simulink model "ImuCalibrator"  (R2018a)
settings: Solver=FixedStepDiscrete  StartTime=0.0  StopTime=inf  FixedStep=1/Fss  RelTol=1e-3
PreLoadFcn:
  | modelDef = getModelDef();
  | Fss = 1;  % nominal IMU sampling rate
  | 
  | gyroCalBiases = [0;0;0];
  | gyroCalMatrix = eye(3);
  | gyroGsensMatrix = zeros(3,3);
  | 
  | accelCalBiases = [0;0;0];
  | accelCalMatrix = eye(3);
  | 
  | imuPar = getImuPar('lmvpUncalibrated');
  | 
  | lastUsedMgyr = zeros(3,3);
undefined symbols (not defined in the file or in its folder): numStates
libraries: simulink x5, vrlib x5, dspinverses x4, dspsigops x2, dspindex x2, dspstat3 x1, simulink_extras x1, dspmtrx3 x1, dspsnks4 x1, dspsrcs4 x1, dspswit3 x1
(part 1 of 2)
settings Model: Creator=Eric  LastModifiedBy=efoxlin
settings OptimizationCC: DefaultParameterBehavior=Inlined  InlineInvariantSignals=on
settings DebuggingCC: UnconnectedOutputMsg=none
settings RTWCC: Toolchain=Microsoft Visual C++ 2017 v15.0 | nmake (64-bit Windows)  BuildConfiguration=Faster Runs
settings GRTTargetCC: MatFileLogging=off  SupportNonFinite=off

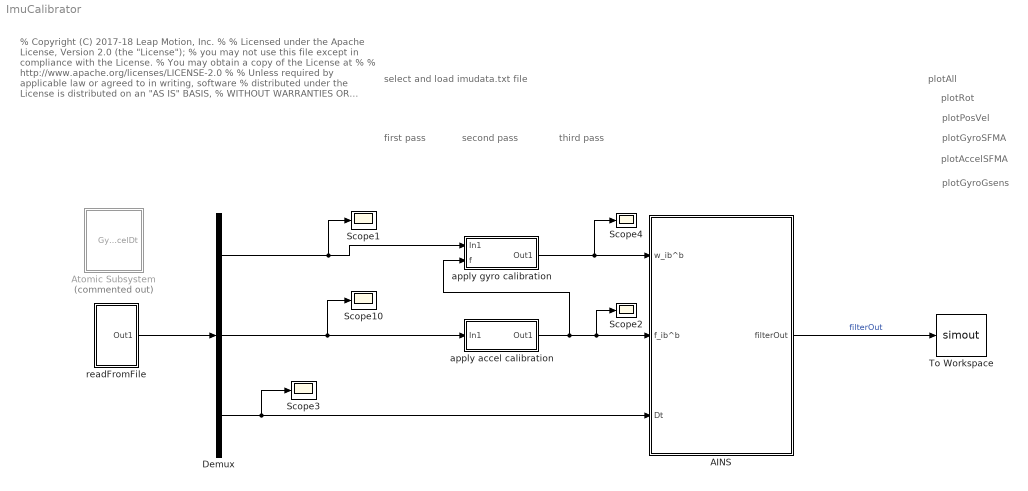
== system ImuCalibrator ==
  note: % Copyright (C) 2017-18 Leap Motion, Inc.
      | %
      | %    Licensed under the Apache License, Version 2.0 (the "License");
      | %    you may not use this file except in compliance with the License.
      | %    You may obtain a copy of the License at
      | %
      | %        http://www.apache.org/licenses/LICENSE-2.0
      | %
      | %    Unless required by applicable law or agreed to in writing, software
      | %    distributed under the License is distributed on an "AS IS" BASIS,
      | %    WITHOUT WARRANTIES OR CONDITIONS OF ANY KIND, either express or implied.
      | %    See the License for the specific language governing permissions and
      | %    limitations under the License.
      | % Author: Eric Foxlin
  note: select and load imudata.txt file
  note: second pass
  note: first pass
  note: plotAccelSFMA
  note: plotGyroSFMA
  note: plotAll
  note: plotPosVel
  note: plotRot
  note: plotGyroGsens
  note: third pass
  AINS : Subsystem  TreatAsAtomicUnit=on
  Atomic Subsystem : Subsystem  Commented=on  TreatAsAtomicUnit=on
  Demux : Demux  Outputs=[3 3 1]
  Scope{1..4,10} (5 alike) : Scope
  To Workspace : ToWorkspace  VariableName=simout  SaveFormat=Timeseries  SampleTime=-1
      settings: Save2DSignal=2-D array (concatenate along first dimension)
  apply accel calibration : Subsystem  TreatAsAtomicUnit=on
  apply gyro calibration : Subsystem  TreatAsAtomicUnit=on
  readFromFile : Subsystem
  wires:
  Demux/3 -> Scope3/1, AINS/3(Dt)
  Demux/2 -> Scope10/1, apply accel calibration/1(In1)
  apply gyro calibration/1(Out1) -> AINS/1(w_ib^b), Scope4/1
  apply accel calibration/1(Out1) -> AINS/2(f_ib^b), Scope2/1, apply gyro calibration/2(f)
  Demux/1 -> apply gyro calibration/1(In1), Scope1/1
  readFromFile/1(Out1) -> Demux/1
  AINS/1(filterOut) -> To Workspace/1  "filterOut"

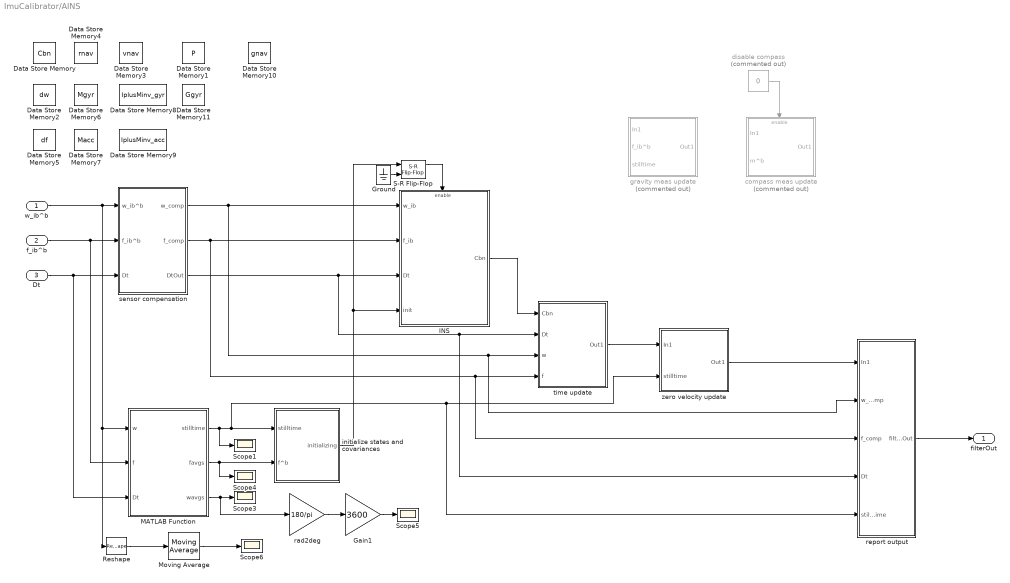
== system ImuCalibrator/AINS ==
  w_ib^b : Inport  Unit=rad/s
  f_ib^b : Inport  Port=2  Unit=m/s^2  PortDimensions=3
  Dt : Inport  Port=3  Unit=rad/s
  Data Store Memory : DataStoreMemory  DataStoreName=Cbn  ReadBeforeWriteMsg=warning  WriteAfterWriteMsg=warning  WriteAfterReadMsg=warning  InitialValue=eye(3)  VectorParams1D=off  ShowAdditionalParam=off
  Data Store Memory1 : DataStoreMemory  DataStoreName=P  ReadBeforeWriteMsg=warning  WriteAfterWriteMsg=warning  WriteAfterReadMsg=warning  InitialValue=eye(modelDef.numStates)*1e-12  ShowAdditionalParam=off
  Data Store Memory10 : DataStoreMemory  DataStoreName=gnav  ReadBeforeWriteMsg=warning  WriteAfterWriteMsg=warning  WriteAfterReadMsg=warning  InitialValue=[0;0; 9.8065]  VectorParams1D=off  ShowAdditionalParam=off
  Data Store Memory11 : DataStoreMemory  DataStoreName=Ggyr  ReadBeforeWriteMsg=warning  WriteAfterWriteMsg=warning  WriteAfterReadMsg=warning  InitialValue=zeros(3,3)  VectorParams1D=off  ShowAdditionalParam=off
  Data Store Memory2 : DataStoreMemory  DataStoreName=dw  ReadBeforeWriteMsg=warning  WriteAfterWriteMsg=warning  WriteAfterReadMsg=warning  InitialValue=[0;0;0]  VectorParams1D=off  ShowAdditionalParam=off
  Data Store Memory3 : DataStoreMemory  DataStoreName=vnav  ReadBeforeWriteMsg=warning  WriteAfterWriteMsg=warning  WriteAfterReadMsg=warning  InitialValue=[0;0;0]  VectorParams1D=off  ShowAdditionalParam=off
  Data Store Memory4 : DataStoreMemory  DataStoreName=rnav  ReadBeforeWriteMsg=warning  WriteAfterWriteMsg=warning  WriteAfterReadMsg=warning  InitialValue=[0;0;0]  VectorParams1D=off  ShowAdditionalParam=off
  Data Store Memory5 : DataStoreMemory  DataStoreName=df  ReadBeforeWriteMsg=warning  WriteAfterWriteMsg=warning  WriteAfterReadMsg=warning  InitialValue=[0;0;0]  VectorParams1D=off  ShowAdditionalParam=off
  Data Store Memory6 : DataStoreMemory  DataStoreName=Mgyr  ReadBeforeWriteMsg=warning  WriteAfterWriteMsg=warning  WriteAfterReadMsg=warning  InitialValue=zeros(3,3)  VectorParams1D=off  ShowAdditionalParam=off
  Data Store Memory7 : DataStoreMemory  DataStoreName=Macc  ReadBeforeWriteMsg=warning  WriteAfterWriteMsg=warning  WriteAfterReadMsg=warning  InitialValue=zeros(3,3)  VectorParams1D=off  ShowAdditionalParam=off
  Data Store Memory8 : DataStoreMemory  DataStoreName=IplusMinv_gyr  ReadBeforeWriteMsg=warning  WriteAfterWriteMsg=warning  WriteAfterReadMsg=warning  InitialValue=eye(3)  VectorParams1D=off  ShowAdditionalParam=off
  Data Store Memory9 : DataStoreMemory  DataStoreName=IplusMinv_acc  ReadBeforeWriteMsg=warning  WriteAfterWriteMsg=warning  WriteAfterReadMsg=warning  InitialValue=eye(3)  VectorParams1D=off  ShowAdditionalParam=off
  Gain1 : Gain  Gain=3600
  Ground : Ground
  INS : Subsystem  Priority=2
  MATLAB Function : MATLAB Function  TreatAsAtomicUnit=on
  Moving Average : dspstat3/Moving Average  Method=Sliding window  ForgettingFactorPort=off  SpecifyWindowLength=on  WindowLength=1000  ForgettingFactor=0.9  SimulateUsing=Code generation
  Reshape : Reshape  OutputDimensionality=Row vector (2-D)
  S-R Flip-Flop : simulink_extras/Flip Flops/S-R Flip-Flop  initial_condition=0
  Scope{1,3..6} (5 alike) : Scope
  compass meas update : Subsystem  Commented=on  TreatAsAtomicUnit=on
  disable compass : Constant  Commented=on  Value=0
  gravity meas update : Subsystem  Commented=on  TreatAsAtomicUnit=on
  initialize states and covariances : Subsystem  Priority=1  TreatAsAtomicUnit=on
  rad2deg : Gain  Gain=180/pi
  report output : Subsystem  Priority=10  TreatAsAtomicUnit=on
  sensor compensation : Subsystem
  time update : Subsystem  Priority=3  TreatAsAtomicUnit=on
  zero velocity update : Subsystem  Priority=4  TreatAsAtomicUnit=on
  filterOut : Outport
  wires:
  time update/1(Out1) -> zero velocity update/1(In1)
  disable compass/1 -> compass meas update/Enable
  MATLAB Function/1(stilltime) -> Scope1/1, report output/5(stilltime), zero velocity update/2(stilltime), initialize states and covariances/1(stilltime)
  MATLAB Function/2(favgs) -> Scope4/1, initialize states and covariances/2(f^b)
  zero velocity update/1(Out1) -> report output/1(In1)
  sensor compensation/1(w_comp) -> report output/2(w_comp), time update/3(w), INS/1(w_ib)
  INS/1(Cbn) -> time update/1(Cbn)
  sensor compensation/3(DtOut) -> report output/4(Dt), time update/2(Dt), INS/3(Dt)
  sensor compensation/2(f_comp) -> INS/2(f_ib), report output/3(f_comp), time update/4(f)
  f_ib^b/1 -> MATLAB Function/2(f), sensor compensation/2(f_ib^b)
  w_ib^b/1 -> MATLAB Function/1(w), Reshape/1, sensor compensation/1(w_ib^b)
  Dt/1 -> MATLAB Function/3(Dt), sensor compensation/3(Dt)
  initialize states and covariances/1(initializing) -> INS/4(init), S-R Flip-Flop/1
  MATLAB Function/3(wavgs) -> rad2deg/1, Scope3/1
  rad2deg/1 -> Gain1/1
  Gain1/1 -> Scope5/1
  Moving Average/1 -> Scope6/1
  Reshape/1 -> Moving Average/1
  S-R Flip-Flop/1 -> INS/Enable
  report output/1(filterOut) -> filterOut/1
  Ground/1 -> S-R Flip-Flop/2

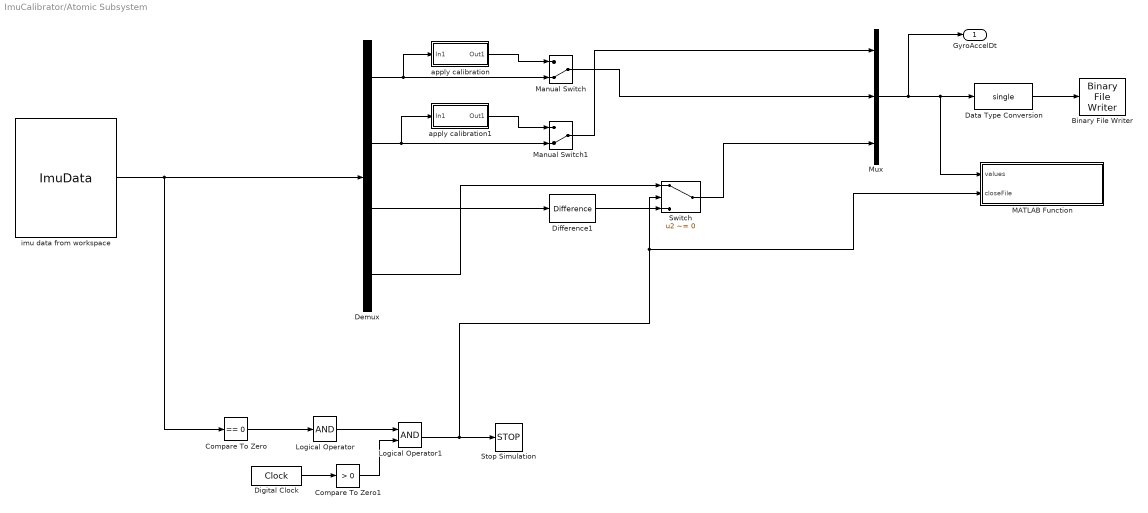
== system ImuCalibrator/Atomic Subsystem ==
  Binary File Writer : dspsnks4/Binary File Writer  Filename=GyroAccelDtFloat32.bin  HeaderStructure=struct([])  SimulateUsing=Code generation
      settings: SourceProductName=DSP System Toolbox  SourceProductBaseCode=DS
  Compare To Zero : simulink/Logic and Bit Operations/Compare To Zero  relop===  OutDataTypeStr=boolean
  Compare To Zero1 : simulink/Logic and Bit Operations/Compare To Zero  relop=>  OutDataTypeStr=boolean
  Data Type Conversion : DataTypeConversion  OutDataTypeStr=single
  Demux : Demux  Outputs=[ 3 3 1 1]
  Difference1 : simulink/Discrete/Difference  ICPrevInput=0.0  OutMin=[]  OutMax=[]  OutDataType=fixdt(1, 16)  OutScaling=2^-10  DoSatur=off
  Digital Clock : DigitalClock  SampleTime=1/Fss
  Logical Operator : Logic  Inputs=1  AllPortsSameDT=off  OutDataTypeStr=boolean
  Logical Operator1 : Logic  AllPortsSameDT=off  OutDataTypeStr=boolean
  MATLAB Function : MATLAB Function  TreatAsAtomicUnit=on
  Manual Switch : ManualSwitch  CurrentSetting=0
  Manual Switch1 : ManualSwitch  CurrentSetting=0
  Mux : Mux  Inputs=[3 3 1]
  Stop Simulation : Stop
  Switch : Switch  Criteria=u2 ~= 0  Threshold=0.5
  apply calibration : Subsystem  TreatAsAtomicUnit=on
  apply calibration1 : Subsystem  TreatAsAtomicUnit=on
  imu data from workspace : FromWorkspace  VariableName=ImuData  SampleTime=1/Fss  Interpolate=off  OutputAfterFinalValue=Setting to zero
  GyroAccelDt : Outport
  wires:
  imu data from workspace/1 -> Compare To Zero/1, Demux/1
  Demux/1 -> Manual Switch/2, apply calibration/1(In1)
  Demux/2 -> Manual Switch1/2, apply calibration1/1(In1)
  Compare To Zero/1 -> Logical Operator/1
  Logical Operator/1 -> Logical Operator1/1
  Manual Switch/1 -> Mux/2
  apply calibration/1(Out1) -> Manual Switch/1
  apply calibration1/1(Out1) -> Manual Switch1/1
  Manual Switch1/1 -> Mux/1
  Logical Operator1/1 -> MATLAB Function/2(closeFile), Switch/2, Stop Simulation/1
  Digital Clock/1 -> Compare To Zero1/1
  Compare To Zero1/1 -> Logical Operator1/2
  Demux/3 -> Difference1/1
  Difference1/1 -> Switch/3
  Switch/1 -> Mux/3
  Demux/4 -> Switch/1
  Mux/1 -> GyroAccelDt/1, MATLAB Function/1(values), Data Type Conversion/1
  Data Type Conversion/1 -> Binary File Writer/1

== system ImuCalibrator/apply accel calibration ==
  In1 : Inport
  Accel SFMA matrix    ameas = M*atrue : Constant  Value=accelCalMatrix  VectorParams1D=off
  "Accel SFMA matrix, column-major1" : Constant  Value="[0.9973\t0.0126\t0.0025\t0.0004\t1.0177\t0.003\t0.0064\t0.0308\t1.0224]"  VectorParams1D=off
  Matrix Multiply : Product  Multiplication=Matrix(*)
  Sum : Sum  Inputs=|+-
  "bias, mg" : Constant  Value=accelCalBiases  VectorParams1D=off
  Out1 : Outport
  wires:
  In1/1 -> Sum/1
  Matrix Multiply/1 -> Out1/1
  Sum/1 -> Matrix Multiply/2
  "bias, mg"/1 -> Sum/2
  Accel SFMA matrix    ameas = M*atrue/1 -> Matrix Multiply/1

== system ImuCalibrator/apply gyro calibration ==
  In1 : Inport
  f : Inport  Port=2
  Accel SFMA matrix    ameas = M*atrue : Constant  Value=gyroCalMatrix  VectorParams1D=off
  Accel SFMA matrix    ameas = M*atrue1 : Constant  Value=gyroGsensMatrix  VectorParams1D=off
  "Accel SFMA matrix, column-major1" : Constant  Value="[0.9973\t0.0126\t0.0025\t0.0004\t1.0177\t0.003\t0.0064\t0.0308\t1.0224]"  VectorParams1D=off
  Matrix Multiply : Product  Multiplication=Matrix(*)
  Matrix Multiply1 : Product  Multiplication=Matrix(*)
  Sum : Sum  Inputs=|+-
  Sum1 : Sum  Inputs=|+-
  "bias, mg" : Constant  Value=gyroCalBiases  VectorParams1D=off
  Out1 : Outport
  wires:
  Accel SFMA matrix    ameas = M*atrue/1 -> Matrix Multiply/1
  "bias, mg"/1 -> Sum/2
  Sum/1 -> Matrix Multiply/2
  Matrix Multiply/1 -> Out1/1
  In1/1 -> Sum1/1
  Sum1/1 -> Sum/1
  Matrix Multiply1/1 -> Sum1/2
  f/1 -> Matrix Multiply1/2
  Accel SFMA matrix    ameas = M*atrue1/1 -> Matrix Multiply1/1

== system ImuCalibrator/readFromFile ==
  Binary File Reader : dspsrcs4/Binary File Reader  Commented=on  Filename=GyroAccelDtFloat32.bin  HeaderStructure=struct([])  DataType=single  SamplesPerFrame=1  IsDataComplex=off  NumChannels=7  OutputEOF=on  SampleTime=1/Fss  SimulateUsing=Code generation
      settings: SourceProductName=DSP System Toolbox  SourceProductBaseCode=DS
  Counter : dspswit3/Counter  Direction=Up  CountEvent=Free running  CounterSize=User defined  MaxCount=4095  InitialCount=0  Output=Hit  HitValue=32  ResetInput=off  SamplesPerFrame=1  Ts=1/Fss  CntDtype=double  HitDtype=Logical
  Data Type Conversion : DataTypeConversion  OutDataTypeStr=double
  MATLAB Function1 : MATLAB Function  Commented=on  TreatAsAtomicUnit=on
  Reshape : Reshape  OutputDimensionality=Column vector (2-D)
  Stop Simulation : Stop
  printTime : Subsystem
  readImuData : Subsystem
  Out1 : Outport
  wires:
  Reshape/1 -> Data Type Conversion/1
  readImuData/1(GyrosAccelsDt) -> Reshape/1
  readImuData/2(EOF) -> Stop Simulation/1
  Data Type Conversion/1 -> Out1/1
  Counter/1 -> printTime/Enable

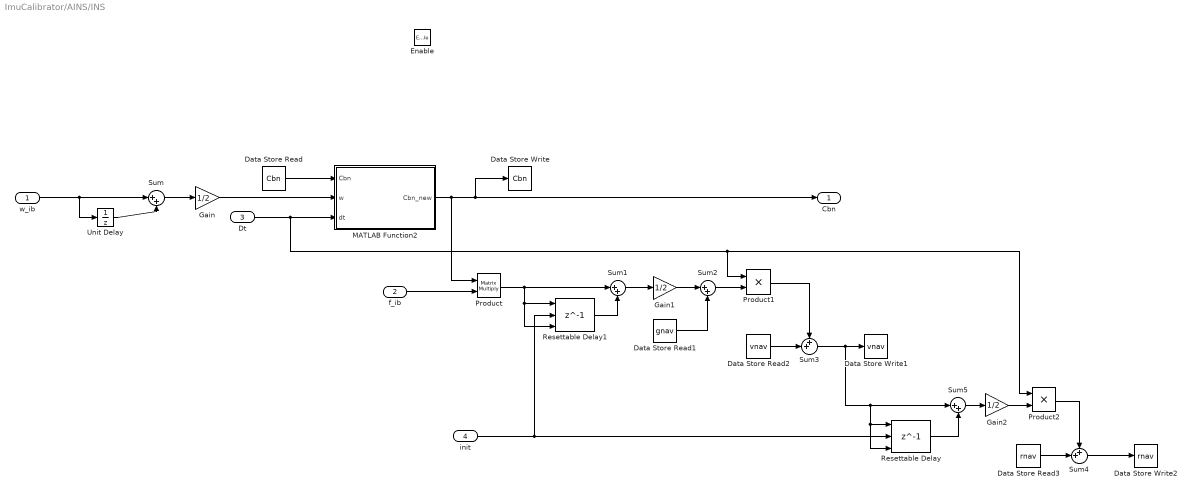
== system ImuCalibrator/AINS/INS ==
  w_ib : Inport
  f_ib : Inport  Port=2
  Dt : Inport  Port=3
  init : Inport  Port=4
  Enable : EnablePort
  Data Store Read : DataStoreRead  DataStoreName=Cbn
  Data Store Read1 : DataStoreRead  DataStoreName=gnav
  Data Store Read2 : DataStoreRead  DataStoreName=vnav
  Data Store Read3 : DataStoreRead  DataStoreName=rnav
  Data Store Write : DataStoreWrite  DataStoreName=Cbn
  Data Store Write1 : DataStoreWrite  DataStoreName=vnav
  Data Store Write2 : DataStoreWrite  DataStoreName=rnav
  Gain : Gain  Gain=1/2
  Gain1 : Gain  Gain=1/2
  Gain2 : Gain  Gain=1/2
  MATLAB Function2 : MATLAB Function  TreatAsAtomicUnit=on
  Product : Product  Multiplication=Matrix(*)
  Product1 : Product
  Product2 : Product
  Resettable Delay : Delay  DelayLength=1  InitialConditionSource=Input port  ExternalReset=Level
      settings: InputPortMap=u0,r5,p4
  Resettable Delay1 : Delay  DelayLength=1  InitialConditionSource=Input port  ExternalReset=Level
      settings: InputPortMap=u0,r5,p4
  Sum{,1..2,5} (4 alike) : Sum  Inputs=|++
  Sum3 : Sum  Inputs=++|
  Sum4 : Sum  Inputs=++|
  Unit Delay : UnitDelay  SampleTime=-1
  Cbn : Outport
  wires:
  Dt/1 -> Product2/1, Product1/1, MATLAB Function2/3(dt)
  Data Store Read/1 -> MATLAB Function2/1(Cbn)
  w_ib/1 -> Unit Delay/1, Sum/1
  MATLAB Function2/1(Cbn_new) -> Product/1, Cbn/1, Data Store Write/1
  Unit Delay/1 -> Sum/2
  Sum/1 -> Gain/1
  Gain/1 -> MATLAB Function2/2(w)
  f_ib/1 -> Product/2
  Data Store Read1/1 -> Sum2/2
  Sum2/1 -> Product1/2
  Product/1 -> Resettable Delay1/3, Resettable Delay1/1, Sum1/1
  Sum1/1 -> Gain1/1
  Gain1/1 -> Sum2/1
  Data Store Read2/1 -> Sum3/2
  Product1/1 -> Sum3/1
  Data Store Read3/1 -> Sum4/2
  Sum4/1 -> Data Store Write2/1
  Sum5/1 -> Gain2/1
  Sum3/1 -> Resettable Delay/3, Resettable Delay/1, Sum5/1, Data Store Write1/1
  Gain2/1 -> Product2/2
  Resettable Delay/1 -> Sum5/2
  init/1 -> Resettable Delay1/2, Resettable Delay/2
  Resettable Delay1/1 -> Sum1/2
  Product2/1 -> Sum4/1

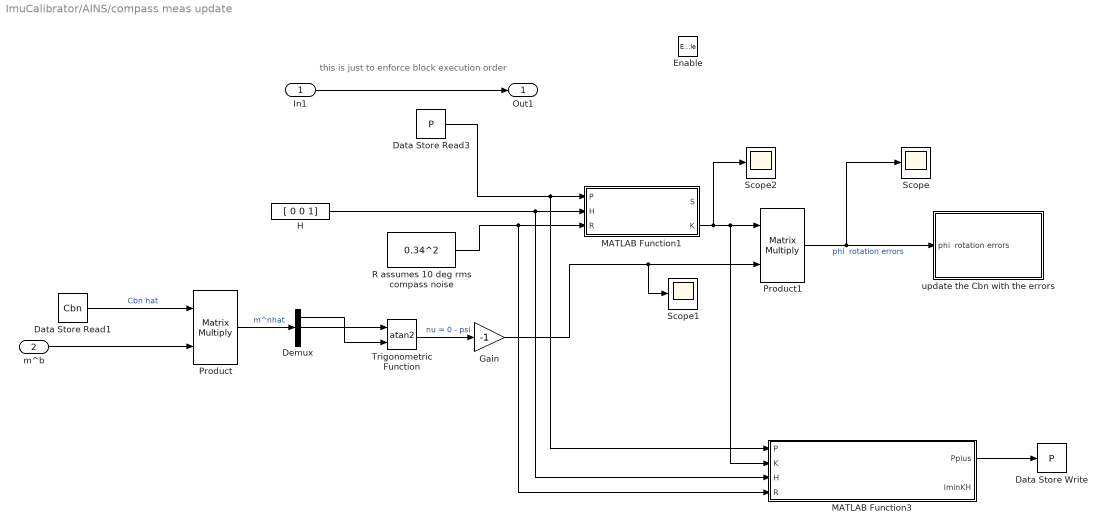
== system ImuCalibrator/AINS/compass meas update ==
  note: this is just to enforce block execution order
  In1 : Inport
  m^b : Inport  Port=2
  Enable : EnablePort
  Data Store Read1 : DataStoreRead  DataStoreName=Cbn
  Data Store Read3 : DataStoreRead  DataStoreName=P
  Data Store Write : DataStoreWrite  DataStoreName=P
  Demux : Demux  Outputs=3
  Gain : Gain  Gain=-1
  H : Constant  Value=[ 0 0 1]  VectorParams1D=off
  MATLAB Function1 : MATLAB Function  TreatAsAtomicUnit=on
  MATLAB Function3 : MATLAB Function  TreatAsAtomicUnit=on
  Product : Product  Multiplication=Matrix(*)
  Product1 : Product  Multiplication=Matrix(*)
  R assumes 10 deg rms compass noise : Constant  Value=0.34^2
  Scope : Scope
  Scope1 : Scope
  Scope2 : Scope
  Trigonometric Function : Trigonometry  Operator=atan2
  update the Cbn with the errors : Subsystem
  Out1 : Outport
  wires:
  Product1/1 -> update the Cbn with the errors/1(phi  rotation errors), Scope/1  "phi  rotation errors"
  R assumes 10 deg rms compass noise/1 -> MATLAB Function1/3(R), MATLAB Function3/4(R)
  Data Store Read3/1 -> MATLAB Function1/1(P), MATLAB Function3/1(P)
  m^b/1 -> Product/2
  MATLAB Function3/1(Pplus) -> Data Store Write/1
  MATLAB Function1/2(K) -> Product1/1, MATLAB Function3/2(K), Scope2/1
  Trigonometric Function/1 -> Gain/1  "nu = 0 - psi"
  Product/1 -> Demux/1  "m^nhat"
  Data Store Read1/1 -> Product/1  "Cbn hat"
  In1/1 -> Out1/1
  Demux/2 -> Trigonometric Function/1
  Demux/1 -> Trigonometric Function/2
  H/1 -> MATLAB Function1/2(H), MATLAB Function3/3(H)
  Gain/1 -> Product1/2, Scope1/1

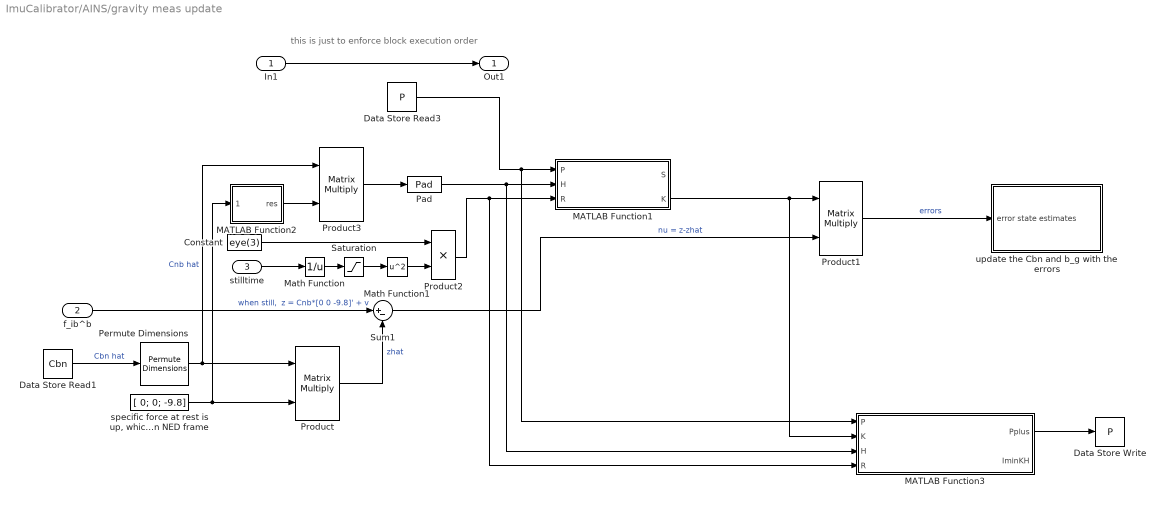
== system ImuCalibrator/AINS/gravity meas update ==
  note: this is just to enforce block execution order
  In1 : Inport
  f_ib^b : Inport  Port=2
  stilltime : Inport  Port=3
  Constant : Constant  Value=eye(3)
  Data Store Read1 : DataStoreRead  DataStoreName=Cbn
  Data Store Read3 : DataStoreRead  DataStoreName=P
  Data Store Write : DataStoreWrite  DataStoreName=P
  MATLAB Function1 : MATLAB Function  TreatAsAtomicUnit=on
  MATLAB Function2 : MATLAB Function  TreatAsAtomicUnit=on
  MATLAB Function3 : MATLAB Function  TreatAsAtomicUnit=on
  Math Function : Math  Operator=reciprocal  SaturateOnIntegerOverflow=on
  Math Function1 : Math  Operator=square  SaturateOnIntegerOverflow=on
  Pad : dspsigops/Pad  padAlong=Rows  dimsToPad=1  valSrc=Specify via dialog  padVal=0  spec=Output size  padNumOutRowsSpecMethod=User-specified  numOutRows=1  padNumOutColsSpecMethod=User-specified  numOutCols=numStates  isVarDimsMode=off  padBeginning=0  padEnd=0  outSizeMode=User-specified  outSize=1  padSigAt=End  trunc_flag=None  roundingMode=Floor  overflowMode=off  truncOrWrapMode=Truncate  wrap_flag=None
      settings: SourceProductName=DSP System Toolbox  SourceProductBaseCode=DS
  Permute Dimensions : PermuteDimensions
  Product : Product  Multiplication=Matrix(*)
  Product1 : Product  Multiplication=Matrix(*)
  Product2 : Product
  Product3 : Product  Multiplication=Matrix(*)
  Saturation : Saturate  UpperLimit=9.8*4  LowerLimit=1
  Sum1 : Sum  Inputs=|+-
  "specific force at rest is up, which is -z in NED frame" : Constant  Value=[ 0; 0; -9.8]
  update the Cbn and b_g with the errors : Subsystem
  Out1 : Outport
  wires:
  In1/1 -> Out1/1
  f_ib^b/1 -> Sum1/1  "when still,  z = Cnb*[0 0 -9.8]' + v"
  Data Store Read1/1 -> Permute Dimensions/1  "Cbn hat"
  Permute Dimensions/1 -> Product3/1, Product/1  "Cnb hat"
  Product/1 -> Sum1/2  "zhat"
  Sum1/1 -> Product1/2  "nu = z-zhat"
  MATLAB Function3/1(Pplus) -> Data Store Write/1
  Product3/1 -> Pad/1
  "specific force at rest is up, which is -z in NED frame"/1 -> MATLAB Function2/1(inp_vr), Product/2
  MATLAB Function2/1(res) -> Product3/2
  Data Store Read3/1 -> MATLAB Function3/1(P), MATLAB Function1/1(P)
  Product2/1 -> MATLAB Function3/4(R), MATLAB Function1/3(R)
  Product1/1 -> update the Cbn and b_g with the errors/1(" error state estimates")  "errors"
  Constant/1 -> Product2/1
  Math Function/1 -> Saturation/1
  Saturation/1 -> Math Function1/1
  stilltime/1 -> Math Function/1
  Math Function1/1 -> Product2/2
  Pad/1 -> MATLAB Function3/3(H), MATLAB Function1/2(H)
  MATLAB Function1/2(K) -> Product1/1, MATLAB Function3/2(K)

== system ImuCalibrator/AINS/initialize states and covariances ==
  stilltime : Inport
  f^b : Inport  Port=2
  Compare To Constant : simulink/Logic and Bit Operations/Compare To Constant  relop=>  const=1.0  OutDataTypeStr=boolean
  Data Store Memory : DataStoreMemory  DataStoreName=INITIALIZED  ReadBeforeWriteMsg=warning  WriteAfterWriteMsg=warning  WriteAfterReadMsg=warning  ShowAdditionalParam=off
  Data Store Read : DataStoreRead  DataStoreName=INITIALIZED
  INITIALIZED = 1 : Subsystem
  Logical Operator : Logic  AllPortsSameDT=off  OutDataTypeStr=boolean
  Logical Operator1 : Logic  Operator=NOT  Inputs=1  IconShape=distinctive  AllPortsSameDT=off  OutDataTypeStr=boolean
  calc Cbn : Subsystem  TreatAsAtomicUnit=on
  set P : Subsystem
  set states : Subsystem  TreatAsAtomicUnit=on
  initializing : Outport
  wires:
  Compare To Constant/1 -> Logical Operator/2
  stilltime/1 -> Compare To Constant/1
  Data Store Read/1 -> Logical Operator1/1
  Logical Operator1/1 -> Logical Operator/1
  f^b/1 -> calc Cbn/1(f^b)
  calc Cbn/2(Cbn) -> set states/1(Cbn)
  INITIALIZED = 1/1(Out1) -> initializing/1
  Logical Operator/1 -> calc Cbn/Enable
  calc Cbn/1(Out1) -> set states/Enable
  set states/1(Out1) -> set P/Enable
  set P/1(Out1) -> INITIALIZED = 1/Enable

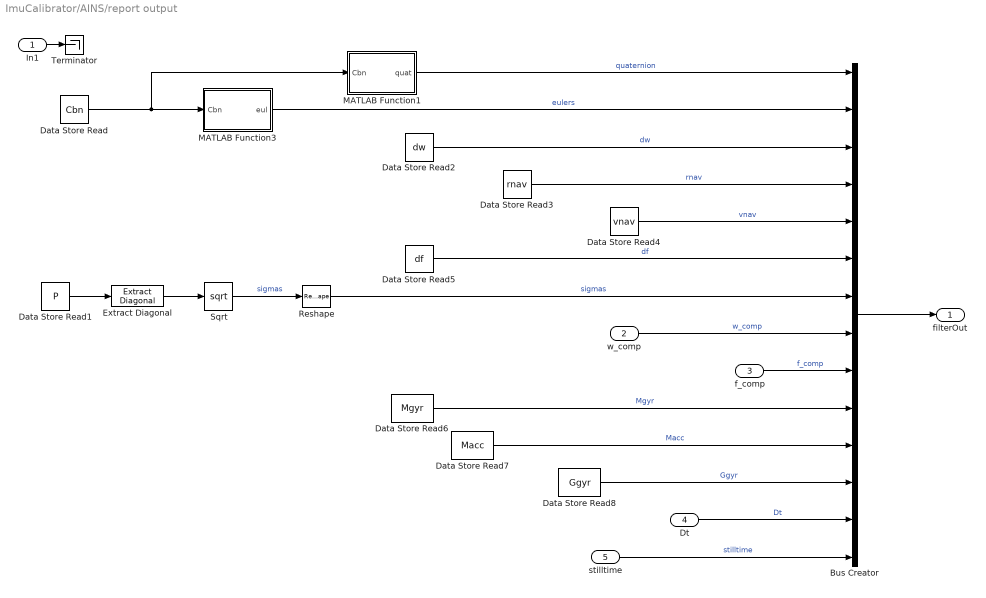
== system ImuCalibrator/AINS/report output ==
  In1 : Inport
  w_comp : Inport  Port=2
  f_comp : Inport  Port=3
  Dt : Inport  Port=4
  stilltime : Inport  Port=5
  Bus Creator : BusCreator  Inputs=14
  Data Store Read : DataStoreRead  DataStoreName=Cbn
  Data Store Read1 : DataStoreRead  DataStoreName=P
  Data Store Read2 : DataStoreRead  DataStoreName=dw
  Data Store Read3 : DataStoreRead  DataStoreName=rnav
  Data Store Read4 : DataStoreRead  DataStoreName=vnav
  Data Store Read5 : DataStoreRead  DataStoreName=df
  Data Store Read6 : DataStoreRead  DataStoreName=Mgyr
  Data Store Read7 : DataStoreRead  DataStoreName=Macc
  Data Store Read8 : DataStoreRead  DataStoreName=Ggyr
  Extract Diagonal : dspmtrx3/Extract Diagonal
      settings: SourceProductName=DSP System Toolbox  SourceProductBaseCode=DS
  MATLAB Function1 : MATLAB Function  TreatAsAtomicUnit=on
  MATLAB Function3 : MATLAB Function  TreatAsAtomicUnit=on
  Reshape : Reshape  OutputDimensionality=Column vector (2-D)
  Sqrt : Sqrt  SaturateOnIntegerOverflow=on
  Terminator : Terminator
  filterOut : Outport
  wires:
  Data Store Read/1 -> MATLAB Function1/1(Cbn), MATLAB Function3/1(Cbn)
  Extract Diagonal/1 -> Sqrt/1
  Data Store Read1/1 -> Extract Diagonal/1
  In1/1 -> Terminator/1
  Bus Creator/1 -> filterOut/1
  Data Store Read6/1 -> Bus Creator/10  "Mgyr"
  Sqrt/1 -> Reshape/1  "sigmas"
  f_comp/1 -> Bus Creator/9  "f_comp"
  Data Store Read8/1 -> Bus Creator/12  "Ggyr"
  Data Store Read5/1 -> Bus Creator/6  "df"
  w_comp/1 -> Bus Creator/8  "w_comp"
  Data Store Read4/1 -> Bus Creator/5  "vnav"
  Data Store Read2/1 -> Bus Creator/3  "dw"
  Data Store Read3/1 -> Bus Creator/4  "rnav"
  MATLAB Function3/1(eul) -> Bus Creator/2  "eulers"
  Data Store Read7/1 -> Bus Creator/11  "Macc"
  MATLAB Function1/1(quat) -> Bus Creator/1  "quaternion"
  Dt/1 -> Bus Creator/13  "Dt"
  stilltime/1 -> Bus Creator/14  "stilltime"
  Reshape/1 -> Bus Creator/7  "sigmas"

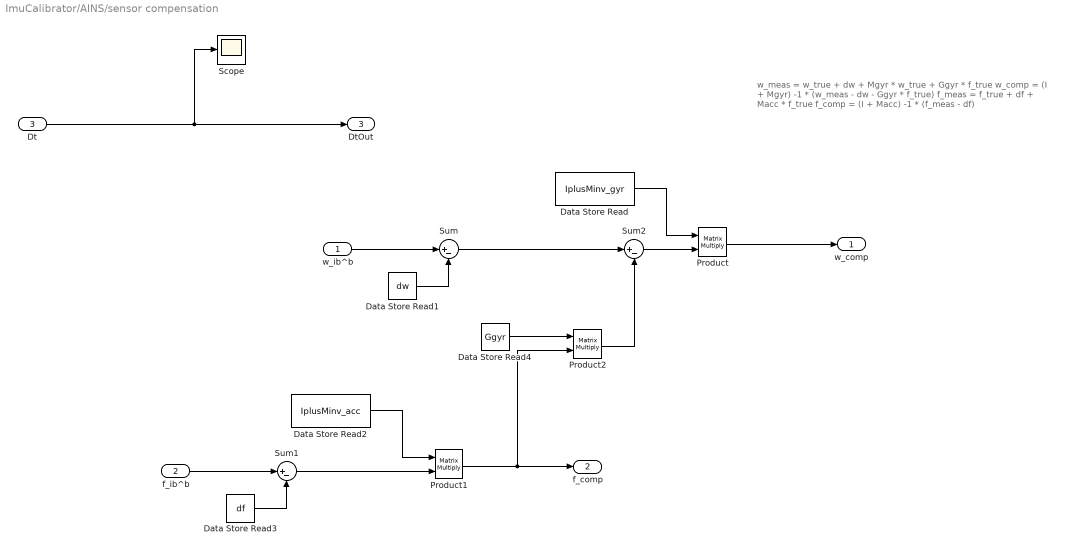
== system ImuCalibrator/AINS/sensor compensation ==
  note: w_meas = w_true + dw + Mgyr * w_true + Ggyr * f_true
      | w_comp = (I + Mgyr) -1 * (w_meas - dw - Ggyr * f_true)
      |
      | f_meas = f_true + df + Macc * f_true
      | f_comp = (I + Macc) -1 * (f_meas - df)
  w_ib^b : Inport  Unit=rad/s
  f_ib^b : Inport  Port=2  Unit=m/s^2  PortDimensions=3
  Dt : Inport  Port=3  Unit=rad/s
  Data Store Read : DataStoreRead  DataStoreName=IplusMinv_gyr
  Data Store Read1 : DataStoreRead  DataStoreName=dw
  Data Store Read2 : DataStoreRead  DataStoreName=IplusMinv_acc
  Data Store Read3 : DataStoreRead  DataStoreName=df
  Data Store Read4 : DataStoreRead  DataStoreName=Ggyr
  Product : Product  Multiplication=Matrix(*)
  Product1 : Product  Multiplication=Matrix(*)
  Product2 : Product  Multiplication=Matrix(*)
  Scope : Scope
  Sum : Sum  Inputs=|+-
  Sum1 : Sum  Inputs=|+-
  Sum2 : Sum  Inputs=|+-
  w_comp : Outport
  f_comp : Outport  Port=2
  DtOut : Outport  Port=3
  wires:
  Dt/1 -> Scope/1, DtOut/1
  Data Store Read1/1 -> Sum/2
  w_ib^b/1 -> Sum/1
  Sum/1 -> Sum2/1
  Data Store Read/1 -> Product/1
  Product/1 -> w_comp/1
  Product1/1 -> Product2/2, f_comp/1
  Data Store Read2/1 -> Product1/1
  Sum1/1 -> Product1/2
  f_ib^b/1 -> Sum1/1
  Data Store Read3/1 -> Sum1/2
  Sum2/1 -> Product/2
  Product2/1 -> Sum2/2
  Data Store Read4/1 -> Product2/1

== system ImuCalibrator/AINS/time update ==
  Cbn : Inport
  Dt : Inport  Port=2
  w : Inport  Port=3
  f : Inport  Port=4
  Constant : Constant  Commented=on  Value=numStates
  Data Store Read : DataStoreRead  DataStoreName=P
  Data Store Read1 : DataStoreRead  DataStoreName=Cbn
  Data Store Write : DataStoreWrite  DataStoreName=P
  MATLAB Function : MATLAB Function  TreatAsAtomicUnit=on
  MATLAB Function1 : MATLAB Function  Commented=on  TreatAsAtomicUnit=on
  MATLAB Function2 : MATLAB Function  Commented=on  TreatAsAtomicUnit=on
  MATLAB Function3 : MATLAB Function  TreatAsAtomicUnit=on
  Permute Dimensions : PermuteDimensions
  Product2 : Product  Inputs=3  Multiplication=Matrix(*)
  Sum : Sum  Inputs=|++
  Out1 : Outport
  wires:
  Cbn/1 -> Out1/1  "this is just to enforce block execution order"
  Dt/1 -> MATLAB Function3/3(Dt), MATLAB Function/3(Dt)
  MATLAB Function3/1(Phi) -> Permute Dimensions/1, Product2/1  "Phi"
  Data Store Read/1 -> Product2/2
  Permute Dimensions/1 -> Product2/3  "Phi'"
  Sum/1 -> Data Store Write/1  "Phi*P*Phi' + Q"
  Data Store Read1/1 -> MATLAB Function3/4(Cbn), MATLAB Function/4(Cbn)
  w/1 -> MATLAB Function3/1(omega), MATLAB Function/1(omega)
  f/1 -> MATLAB Function3/2(fbod), MATLAB Function/2(f_ib)
  Constant/1 -> MATLAB Function2/1(numStates)
  MATLAB Function/1(Q) -> Sum/2
  Product2/1 -> Sum/1  "Phi*P*Phi'"

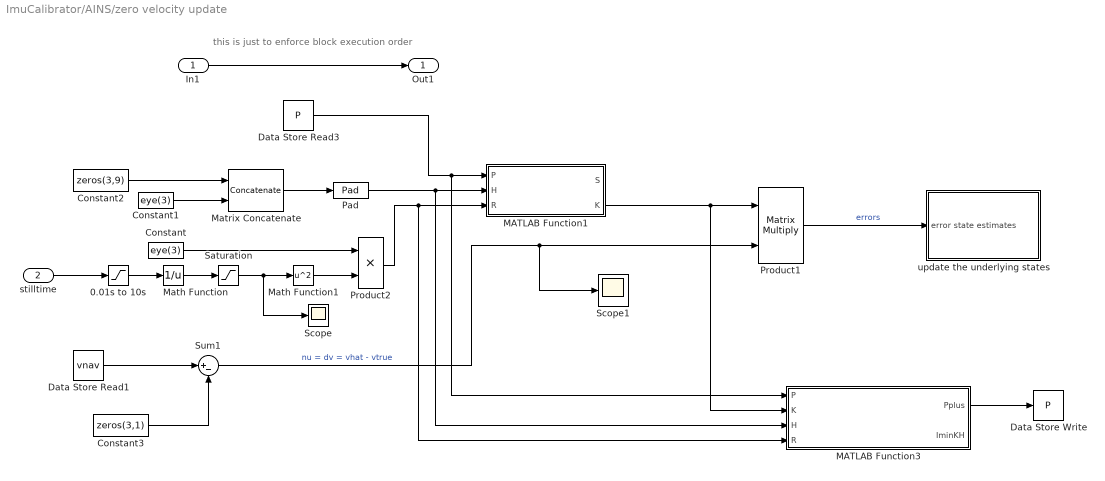
== system ImuCalibrator/AINS/zero velocity update ==
  note: this is just to enforce block execution order
  In1 : Inport
  stilltime : Inport  Port=2
  0.01s to 10s : Saturate  UpperLimit=10  LowerLimit=0.01
  Constant : Constant  Value=eye(3)
  Constant1 : Constant  Value=eye(3)
  Constant2 : Constant  Value=zeros(3,9)  VectorParams1D=off
  Constant3 : Constant  Value=zeros(3,1)  VectorParams1D=off
  Data Store Read1 : DataStoreRead  DataStoreName=vnav
  Data Store Read3 : DataStoreRead  DataStoreName=P
  Data Store Write : DataStoreWrite  DataStoreName=P
  MATLAB Function1 : MATLAB Function  TreatAsAtomicUnit=on
  MATLAB Function3 : MATLAB Function  TreatAsAtomicUnit=on
  Math Function : Math  Operator=reciprocal  SaturateOnIntegerOverflow=on
  Math Function1 : Math  Operator=square  SaturateOnIntegerOverflow=on
  Matrix Concatenate : Concatenate  Mode=Multidimensional array  ConcatenateDimension=2
  Pad : dspsigops/Pad  padAlong=Rows  dimsToPad=1  valSrc=Specify via dialog  padVal=0  spec=Output size  padNumOutRowsSpecMethod=User-specified  numOutRows=1  padNumOutColsSpecMethod=User-specified  numOutCols=modelDef.numStates  isVarDimsMode=off  padBeginning=0  padEnd=0  outSizeMode=User-specified  outSize=1  padSigAt=End  trunc_flag=None  roundingMode=Floor  overflowMode=off  truncOrWrapMode=Truncate  wrap_flag=None
      settings: SourceProductName=DSP System Toolbox  SourceProductBaseCode=DS
  Product1 : Product  Multiplication=Matrix(*)
  Product2 : Product
  Saturation : Saturate  UpperLimit=100  LowerLimit=0.1
  Scope : Scope
  Scope1 : Scope
  Sum1 : Sum  Inputs=|+-
  update the underlying states : Subsystem
  Out1 : Outport
  wires:
  MATLAB Function1/2(K) -> Product1/1, MATLAB Function3/2(K)
  Pad/1 -> MATLAB Function1/2(H), MATLAB Function3/3(H)
  Math Function1/1 -> Product2/2
  stilltime/1 -> 0.01s to 10s/1
  Saturation/1 -> Scope/1, Math Function1/1
  Math Function/1 -> Saturation/1
  Constant/1 -> Product2/1
  Product1/1 -> update the underlying states/1(" error state estimates")  "errors"
  Product2/1 -> MATLAB Function1/3(R), MATLAB Function3/4(R)
  Data Store Read3/1 -> MATLAB Function1/1(P), MATLAB Function3/1(P)
  Matrix Concatenate/1 -> Pad/1
  MATLAB Function3/1(Pplus) -> Data Store Write/1
  Sum1/1 -> Scope1/1, Product1/2  "nu = dv = vhat - vtrue"
  In1/1 -> Out1/1
  Constant2/1 -> Matrix Concatenate/1
  Constant1/1 -> Matrix Concatenate/2
  0.01s to 10s/1 -> Math Function/1
  Data Store Read1/1 -> Sum1/1
  Constant3/1 -> Sum1/2

== system ImuCalibrator/Atomic Subsystem/apply calibration ==
  In1 : Inport
  " LU Inverse" : dspinverses/ LU Inverse
      settings: SourceProductName=DSP System Toolbox
  Accel SFMA matrix    ameas = M*atrue : Constant  Value="[1.0015  -0.001 0.006;  0.004 1.0025 0.021; -0.01 -0.02 1.0096]"  VectorParams1D=off
  "Accel SFMA matrix, column-major1" : Constant  Value="[0.9973\t0.0126\t0.0025\t0.0004\t1.0177\t0.003\t0.0064\t0.0308\t1.0224]"  VectorParams1D=off
  Matrix Multiply : Product  Multiplication=Matrix(*)
  Scope1 : Scope
  Scope10 : Scope
  Scope2 : Scope
  Sum : Sum  Inputs=|+-
  "bias, mg" : Constant  Value="[0.035;\t-0.125;\t-0.15]"  VectorParams1D=off
  "bias, mg1" : Constant  Value="[2.63054;\t-11.1493;\t-13.6156]"  VectorParams1D=off
  Out1 : Outport
  wires:
  In1/1 -> Scope10/1, Sum/1
  Accel SFMA matrix    ameas = M*atrue/1 -> " LU Inverse"/1
  Matrix Multiply/1 -> Scope2/1, Out1/1
  Sum/1 -> Scope1/1, Matrix Multiply/2
  "bias, mg"/1 -> Sum/2
  " LU Inverse"/1 -> Matrix Multiply/1

== system ImuCalibrator/Atomic Subsystem/apply calibration1 ==
  In1 : Inport
  " LU Inverse" : dspinverses/ LU Inverse
      settings: SourceProductName=DSP System Toolbox
  Gain : Gain  Gain=pi/180
  "Gyro SFMA matrix, column-major" : Constant  Value="[1.0176\t-0.0073\t0.0116\t0.0026\t1.0207\t0.0199\t0.0223\t-0.0243\t1.0377\t]"  VectorParams1D=off
  Matrix Multiply : Product  Multiplication=Matrix(*)
  Permute Dimensions : PermuteDimensions
  Reshape : Reshape  OutputDimensionality=Customize  OutputDimensions=[3,3]
  Scope1 : Scope
  Scope10 : Scope
  Scope2 : Scope
  Sum : Sum  Inputs=|+-
  bias,deg/s : Constant  Value="[-0.36096;\t0.27502;\t0.171887]"  VectorParams1D=off
  Out1 : Outport
  wires:
  In1/1 -> Scope10/1, Sum/1
  "Gyro SFMA matrix, column-major"/1 -> Reshape/1
  Reshape/1 -> Permute Dimensions/1
  Permute Dimensions/1 -> " LU Inverse"/1
  Matrix Multiply/1 -> Scope2/1, Out1/1
  bias,deg/s/1 -> Gain/1
  Sum/1 -> Scope1/1, Matrix Multiply/2
  Gain/1 -> Sum/2
  " LU Inverse"/1 -> Matrix Multiply/1

== system ImuCalibrator/readFromFile/printTime ==
  Enable : EnablePort
  Digital Clock : DigitalClock  SampleTime=1/Fss
  MATLAB Function : MATLAB Function  TreatAsAtomicUnit=on
  wires:
  Digital Clock/1 -> MATLAB Function/1(u)

== system ImuCalibrator/readFromFile/readImuData ==
  C++ S-function : S-Function  FunctionName=readImuData  Parameters=1/Fss  SFunctionDeploymentMode=off  EnableBusSupport=off
  Constant : Constant  Value=0
  Constant1 : Constant
  Difference : simulink/Discrete/Difference  ICPrevInput=0.0  OutMin=[]  OutMax=[]  OutDataType=fixdt(1, 16)  OutScaling=2^-10  DoSatur=off
  Mux : Mux  Inputs=2
  Terminator : Terminator
  Unit Delay : UnitDelay  SampleTime=-1
  Unit Delay1 : UnitDelay  SampleTime=-1
  avoid huge jump on first cycle : Switch  Criteria=u2 > Threshold  Threshold=0.5
  avoid sending garbage on the last row : Switch  Criteria=u2 > Threshold  Threshold=0.5
  gyros accels : Selector  InputPortWidth=11  IndexOptions=Index vector (dialog)  Indices=[5:10]  OutputSizes=1
  tstamp : Selector  InputPortWidth=11  IndexOptions=Index vector (dialog)  Indices=3  OutputSizes=1
  GyrosAccelsDt : Outport
  EOF : Outport  Port=2
  wires:
  C++ S-function/2 -> avoid sending garbage on the last row/2, EOF/1
  tstamp/1 -> Difference/1
  C++ S-function/1 -> gyros accels/1, tstamp/1
  gyros accels/1 -> Mux/1
  Mux/1 -> Unit Delay/1, avoid sending garbage on the last row/3
  Difference/1 -> avoid huge jump on first cycle/1
  avoid sending garbage on the last row/1 -> GyrosAccelsDt/1
  Unit Delay/1 -> avoid sending garbage on the last row/1
  avoid huge jump on first cycle/1 -> Mux/2
  Constant/1 -> avoid huge jump on first cycle/3
  Unit Delay1/1 -> avoid huge jump on first cycle/2
  Constant1/1 -> Unit Delay1/1
  C++ S-function/3 -> Terminator/1

== system ImuCalibrator/AINS/compass meas update/update the Cbn with the errors ==
  phi  rotation errors : Inport
  Data Store Read2 : DataStoreRead  DataStoreName=Cbn
  Data Store Write1 : DataStoreWrite  DataStoreName=Cbn
  MATLAB Function : MATLAB Function  TreatAsAtomicUnit=on
  Product2 : Product  Multiplication=Matrix(*)
  Sum : Sum  Inputs=++|
  re-orthonormalization : Subsystem  TreatAsAtomicUnit=on
  wires:
  re-orthonormalization/1(Out1) -> Data Store Write1/1
  Data Store Read2/1 -> Sum/2, Product2/2
  phi  rotation errors/1 -> MATLAB Function/1(inp_vr)
  Sum/1 -> re-orthonormalization/1(In1)
  Product2/1 -> Sum/1
  MATLAB Function/1(res) -> Product2/1  "[phi X]"

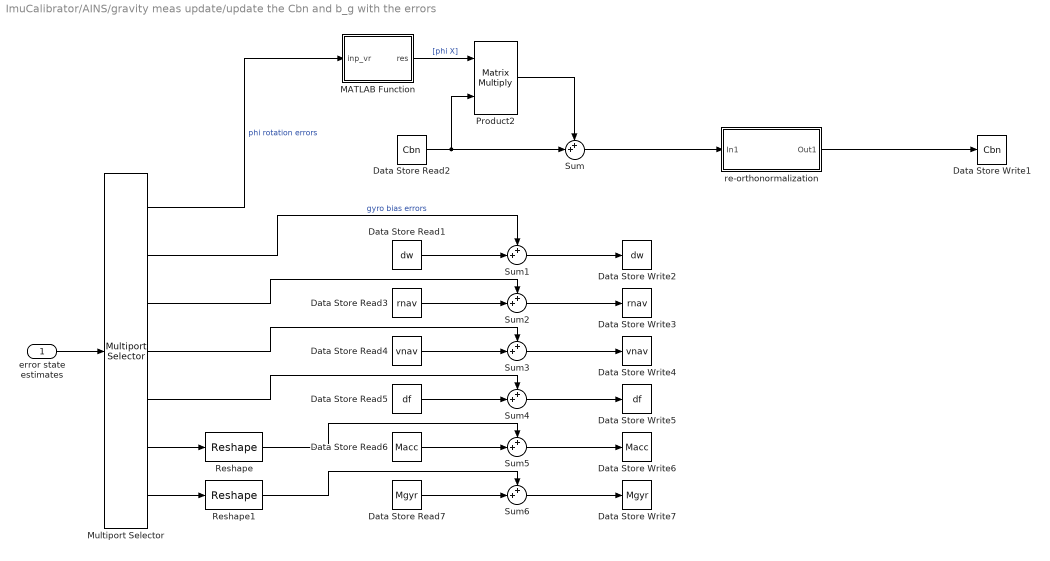
== system ImuCalibrator/AINS/gravity meas update/update the Cbn and b_g with the errors ==
  " error state estimates" : Inport
  Data Store Read1 : DataStoreRead  DataStoreName=dw
  Data Store Read2 : DataStoreRead  DataStoreName=Cbn
  Data Store Read3 : DataStoreRead  DataStoreName=rnav
  Data Store Read4 : DataStoreRead  DataStoreName=vnav
  Data Store Read5 : DataStoreRead  DataStoreName=df
  Data Store Read6 : DataStoreRead  DataStoreName=Macc
  Data Store Read7 : DataStoreRead  DataStoreName=Mgyr
  Data Store Write1 : DataStoreWrite  DataStoreName=Cbn
  Data Store Write2 : DataStoreWrite  DataStoreName=dw
  Data Store Write3 : DataStoreWrite  DataStoreName=rnav
  Data Store Write4 : DataStoreWrite  DataStoreName=vnav
  Data Store Write5 : DataStoreWrite  DataStoreName=df
  Data Store Write6 : DataStoreWrite  DataStoreName=Macc
  Data Store Write7 : DataStoreWrite  DataStoreName=Mgyr
  MATLAB Function : MATLAB Function  TreatAsAtomicUnit=on
  Multiport Selector : dspindex/Multiport Selector  rowsOrCols=Rows  idxCellArray={ 1:3, 4:6, 7:9, 10:12, 13:15, 16:24, 25:33 }  idxErrMode=Clip Index
  Product2 : Product  Multiplication=Matrix(*)
  Reshape : Reshape  OutputDimensionality=Customize  OutputDimensions=[3,3]
  Reshape1 : Reshape  OutputDimensionality=Customize  OutputDimensions=[3,3]
  Sum{,1..6} (7 alike) : Sum  Inputs=++|
  re-orthonormalization : Subsystem  TreatAsAtomicUnit=on
  wires:
  MATLAB Function/1(res) -> Product2/1  "[phi X]"
  Product2/1 -> Sum/1
  Sum/1 -> re-orthonormalization/1(In1)
  Data Store Read2/1 -> Product2/2, Sum/2
  re-orthonormalization/1(Out1) -> Data Store Write1/1
  Multiport Selector/1 -> MATLAB Function/1(inp_vr)  "phi rotation errors"
  Data Store Read1/1 -> Sum1/2
  Sum1/1 -> Data Store Write2/1
  Multiport Selector/2 -> Sum1/1  "gyro bias errors"
  " error state estimates"/1 -> Multiport Selector/1
  Sum2/1 -> Data Store Write3/1
  Data Store Read3/1 -> Sum2/2
  Data Store Read4/1 -> Sum3/2
  Sum3/1 -> Data Store Write4/1
  Multiport Selector/3 -> Sum2/1
  Multiport Selector/4 -> Sum3/1
  Sum4/1 -> Data Store Write5/1
  Data Store Read5/1 -> Sum4/2
  Multiport Selector/5 -> Sum4/1
  Data Store Read6/1 -> Sum5/2
  Sum5/1 -> Data Store Write6/1
  Sum6/1 -> Data Store Write7/1
  Data Store Read7/1 -> Sum6/2
  Multiport Selector/6 -> Reshape/1
  Reshape/1 -> Sum5/1
  Multiport Selector/7 -> Reshape1/1
  Reshape1/1 -> Sum6/1

== system ImuCalibrator/AINS/initialize states and covariances/INITIALIZED = 1 ==
  Enable : EnablePort  ShowOutputPort=on
  Constant : Constant
  Data Store Write : DataStoreWrite  DataStoreName=INITIALIZED
  Out1 : Outport  OutputWhenDisabled=reset  InitialOutput=false
  wires:
  Constant/1 -> Data Store Write/1
  Enable/1 -> Out1/1

== system ImuCalibrator/AINS/initialize states and covariances/calc Cbn ==
  f^b : Inport
  Enable : EnablePort  ShowOutputPort=on
  Constant : Constant  Value=[1 0 0]
  Cross Product : vrlib/Utilities/Cross Product
      settings: SourceProductBaseCode=VR
  Cross Product1 : vrlib/Utilities/Cross Product
      settings: SourceProductBaseCode=VR
  Gain : Gain  Gain=-1
  Matrix Concatenate : Concatenate  NumInputs=3  Mode=Multidimensional array
  Normalize Vector : vrlib/Utilities/Normalize Vector  maxzero=0
      settings: SourceProductName=Simulink 3D Animation  SourceProductBaseCode=VR
  Normalize Vector1 : vrlib/Utilities/Normalize Vector  maxzero=0
      settings: SourceProductName=Simulink 3D Animation  SourceProductBaseCode=VR
  Normalize Vector2 : vrlib/Utilities/Normalize Vector  maxzero=0
      settings: SourceProductName=Simulink 3D Animation  SourceProductBaseCode=VR
  Out1 : Outport  OutputWhenDisabled=reset  InitialOutput=false
  Cbn : Outport  Port=2
  wires:
  f^b/1 -> Gain/1  "up"
  Gain/1 -> Normalize Vector2/1, Cross Product1/2, Cross Product/1  "down^b"
  Constant/1 -> Cross Product/2
  Cross Product/1 -> Normalize Vector1/1, Cross Product1/1  "east^b"
  Cross Product1/1 -> Normalize Vector/1  "north^b"
  Normalize Vector/1 -> Matrix Concatenate/1
  Normalize Vector1/1 -> Matrix Concatenate/2
  Normalize Vector2/1 -> Matrix Concatenate/3
  Matrix Concatenate/1 -> Cbn/1
  Enable/1 -> Out1/1

== system ImuCalibrator/AINS/initialize states and covariances/set P ==
  Enable : EnablePort  ShowOutputPort=on
  Data Store Write : DataStoreWrite  DataStoreName=P
  Gain : Gain
  Gain2 : Gain
  Gain3 : Gain
  MATLAB Function1 : MATLAB Function  TreatAsAtomicUnit=on
  "initial position error, m rms" : Constant  Value=[0.01; 0.01; 0.01]  VectorParams1D=off
  "initial rotation error, rad rms" : Constant  Value=[0.1; 0.1; 0.1]  VectorParams1D=off
  "initial vel error, m/s" : Constant  Value=[0.01; 0.01; 0.01]  VectorParams1D=off
  Out1 : Outport  OutputWhenDisabled=reset  InitialOutput=false
  wires:
  MATLAB Function1/1(P0) -> Data Store Write/1
  "initial rotation error, rad rms"/1 -> Gain/1
  "initial position error, m rms"/1 -> Gain2/1
  Gain/1 -> MATLAB Function1/1(initialRotUncert)
  Gain2/1 -> MATLAB Function1/2(initialPosUncert)
  "initial vel error, m/s"/1 -> Gain3/1
  Gain3/1 -> MATLAB Function1/3(initialVelUncert)
  Enable/1 -> Out1/1

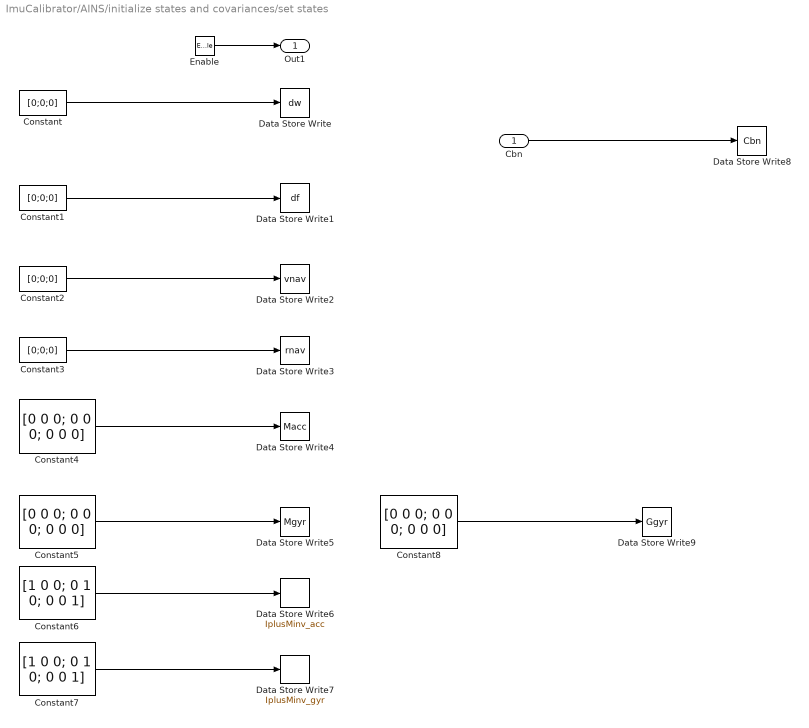
== system ImuCalibrator/AINS/initialize states and covariances/set states ==
  Cbn : Inport
  Enable : EnablePort  ShowOutputPort=on
  Constant{,1..3} (4 alike) : Constant  Value=[0;0;0]
  Constant4 : Constant  Value=[0 0 0; 0 0 0; 0 0 0]  VectorParams1D=off
  Constant5 : Constant  Value=[0 0 0; 0 0 0; 0 0 0]  VectorParams1D=off
  Constant6 : Constant  Value=[1 0 0; 0 1 0; 0 0 1]  VectorParams1D=off
  Constant7 : Constant  Value=[1 0 0; 0 1 0; 0 0 1]  VectorParams1D=off
  Constant8 : Constant  Value=[0 0 0; 0 0 0; 0 0 0]  VectorParams1D=off
  Data Store Write : DataStoreWrite  DataStoreName=dw
  Data Store Write1 : DataStoreWrite  DataStoreName=df
  Data Store Write2 : DataStoreWrite  DataStoreName=vnav
  Data Store Write3 : DataStoreWrite  DataStoreName=rnav
  Data Store Write4 : DataStoreWrite  DataStoreName=Macc
  Data Store Write5 : DataStoreWrite  DataStoreName=Mgyr
  Data Store Write6 : DataStoreWrite  DataStoreName=IplusMinv_acc
  Data Store Write7 : DataStoreWrite  DataStoreName=IplusMinv_gyr
  Data Store Write8 : DataStoreWrite  DataStoreName=Cbn
  Data Store Write9 : DataStoreWrite  DataStoreName=Ggyr
  Out1 : Outport  OutputWhenDisabled=reset  InitialOutput=false
  wires:
  Constant/1 -> Data Store Write/1
  Constant1/1 -> Data Store Write1/1
  Constant2/1 -> Data Store Write2/1
  Constant3/1 -> Data Store Write3/1
  Constant4/1 -> Data Store Write4/1
  Constant5/1 -> Data Store Write5/1
  Constant6/1 -> Data Store Write6/1
  Constant7/1 -> Data Store Write7/1
  Enable/1 -> Out1/1
  Cbn/1 -> Data Store Write8/1
  Constant8/1 -> Data Store Write9/1

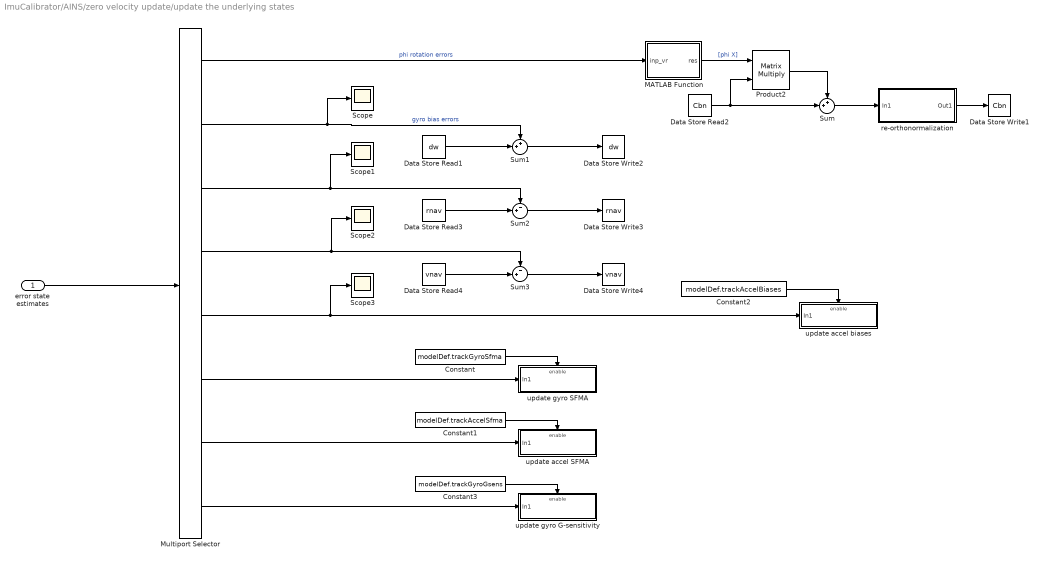
== system ImuCalibrator/AINS/zero velocity update/update the underlying states ==
  " error state estimates" : Inport
  Constant : Constant  Value=modelDef.trackGyroSfma
  Constant1 : Constant  Value=modelDef.trackAccelSfma
  Constant2 : Constant  Value=modelDef.trackAccelBiases
  Constant3 : Constant  Value=modelDef.trackGyroGsens
  Data Store Read1 : DataStoreRead  DataStoreName=dw
  Data Store Read2 : DataStoreRead  DataStoreName=Cbn
  Data Store Read3 : DataStoreRead  DataStoreName=rnav
  Data Store Read4 : DataStoreRead  DataStoreName=vnav
  Data Store Write1 : DataStoreWrite  DataStoreName=Cbn
  Data Store Write2 : DataStoreWrite  DataStoreName=dw
  Data Store Write3 : DataStoreWrite  DataStoreName=rnav
  Data Store Write4 : DataStoreWrite  DataStoreName=vnav
  MATLAB Function : MATLAB Function  TreatAsAtomicUnit=on
  Multiport Selector : dspindex/Multiport Selector  rowsOrCols=Rows  idxCellArray={ 1:3, 4:6, 7:9, 10:12, 13:15, 16:24, 25:33, 34:42 }  idxErrMode=Clip Index
  Product2 : Product  Multiplication=Matrix(*)
  Scope{,1..3} (4 alike) : Scope
  Sum : Sum  Inputs=++|
  Sum1 : Sum  Inputs=++|
  Sum2 : Sum  Inputs=-+|
  Sum3 : Sum  Inputs=-+|
  re-orthonormalization : Subsystem  TreatAsAtomicUnit=on
  update accel SFMA : Subsystem
  update accel biases : Subsystem
  update gyro G-sensitivity : Subsystem
  update gyro SFMA : Subsystem
  wires:
  Multiport Selector/4 -> Sum3/1, Scope2/1
  Multiport Selector/3 -> Sum2/1, Scope1/1
  Sum3/1 -> Data Store Write4/1
  Data Store Read4/1 -> Sum3/2
  Data Store Read3/1 -> Sum2/2
  Sum2/1 -> Data Store Write3/1
  " error state estimates"/1 -> Multiport Selector/1
  Multiport Selector/2 -> Sum1/1, Scope/1  "gyro bias errors"
  Sum1/1 -> Data Store Write2/1
  Data Store Read1/1 -> Sum1/2
  Multiport Selector/1 -> MATLAB Function/1(inp_vr)  "phi rotation errors"
  re-orthonormalization/1(Out1) -> Data Store Write1/1
  Data Store Read2/1 -> Sum/2, Product2/2
  Sum/1 -> re-orthonormalization/1(In1)
  Product2/1 -> Sum/1
  MATLAB Function/1(res) -> Product2/1  "[phi X]"
  Constant/1 -> update gyro SFMA/Enable
  Multiport Selector/6 -> update gyro SFMA/1(In1)
  Constant1/1 -> update accel SFMA/Enable
  Multiport Selector/7 -> update accel SFMA/1(In1)
  Multiport Selector/5 -> update accel biases/1(In1), Scope3/1
  Constant2/1 -> update accel biases/Enable
  Constant3/1 -> update gyro G-sensitivity/Enable
  Multiport Selector/8 -> update gyro G-sensitivity/1(In1)

== system ImuCalibrator/AINS/compass meas update/update the Cbn with the errors/re-orthonormalization ==
  note: Cfixed = C + 0.5(I-CC')C
  note: from http://www.dtic.mil/dtic/tr/fulltext/u2/p003621.pdf page 12
  In1 : Inport
  C*C' : Product  Multiplication=Matrix(*)
  C*C'1 : Product  Multiplication=Matrix(*)
  Constant : Constant  Value=eye(3)
  Display : Display
  Gain : Gain  Gain=1/2
  Permute Dimensions : PermuteDimensions
  Sum : Sum  Inputs=|++
  Sum1 : Sum  Inputs=|+-
  Out1 : Outport
  wires:
  C*C'1/1 -> Gain/1
  Sum1/1 -> C*C'1/1
  Gain/1 -> Sum/2
  Constant/1 -> Sum1/1
  C*C'/1 -> Sum1/2
  Permute Dimensions/1 -> C*C'/2
  Sum/1 -> Out1/1, Display/1
  In1/1 -> Sum/1, C*C'1/2, C*C'/1, Permute Dimensions/1

== system ImuCalibrator/AINS/gravity meas update/update the Cbn and b_g with the errors/re-orthonormalization ==
  note: from http://www.dtic.mil/dtic/tr/fulltext/u2/p003621.pdf page 12
  note: Cfixed = C + 0.5(I-CC')C
  In1 : Inport
  C*C' : Product  Multiplication=Matrix(*)
  C*C'1 : Product  Multiplication=Matrix(*)
  Constant : Constant  Value=eye(3)
  Gain : Gain  Gain=1/2
  Permute Dimensions : PermuteDimensions
  Sum : Sum  Inputs=|++
  Sum1 : Sum  Inputs=|+-
  Out1 : Outport
  wires:
  In1/1 -> Permute Dimensions/1, C*C'/1, C*C'1/2, Sum/1
  Sum/1 -> Out1/1
  Permute Dimensions/1 -> C*C'/2
  C*C'/1 -> Sum1/2
  Constant/1 -> Sum1/1
  Gain/1 -> Sum/2
  Sum1/1 -> C*C'1/1
  C*C'1/1 -> Gain/1

== system ImuCalibrator/AINS/zero velocity update/update the underlying states/re-orthonormalization ==
  note: Cfixed = C + 0.5(I-CC')C
  note: from http://www.dtic.mil/dtic/tr/fulltext/u2/p003621.pdf page 12
  In1 : Inport
  C*C' : Product  Multiplication=Matrix(*)
  C*C'1 : Product  Multiplication=Matrix(*)
  Constant : Constant  Value=eye(3)
  Gain : Gain  Gain=1/2
  Permute Dimensions : PermuteDimensions
  Sum : Sum  Inputs=|++
  Sum1 : Sum  Inputs=|+-
  Out1 : Outport
  wires:
  C*C'1/1 -> Gain/1
  Sum1/1 -> C*C'1/1
  Gain/1 -> Sum/2
  Constant/1 -> Sum1/1
  C*C'/1 -> Sum1/2
  Permute Dimensions/1 -> C*C'/2
  Sum/1 -> Out1/1
  In1/1 -> Sum/1, C*C'1/2, C*C'/1, Permute Dimensions/1

== system ImuCalibrator/AINS/zero velocity update/update the underlying states/update accel SFMA ==
  In1 : Inport
  Enable : EnablePort
  " LU Inverse" : dspinverses/ LU Inverse
      settings: SourceProductName=DSP System Toolbox
  Bias : Bias  Bias=eye(3)
  Data Store Read6 : DataStoreRead  DataStoreName=Macc
  Data Store Write6 : DataStoreWrite  DataStoreName=Macc
  Data Store Write9 : DataStoreWrite  DataStoreName=IplusMinv_acc
  Reshape : Reshape  OutputDimensionality=Customize  OutputDimensions=[3,3]
  Sum5 : Sum  Inputs=++|
  wires:
  Sum5/1 -> Bias/1, Data Store Write6/1
  Data Store Read6/1 -> Sum5/2
  Reshape/1 -> Sum5/1
  In1/1 -> Reshape/1
  Bias/1 -> " LU Inverse"/1
  " LU Inverse"/1 -> Data Store Write9/1

== system ImuCalibrator/AINS/zero velocity update/update the underlying states/update accel biases ==
  In1 : Inport
  Enable : EnablePort
  Data Store Read5 : DataStoreRead  DataStoreName=df
  Data Store Write5 : DataStoreWrite  DataStoreName=df
  Sum4 : Sum  Inputs=++|
  wires:
  Sum4/1 -> Data Store Write5/1
  Data Store Read5/1 -> Sum4/2
  In1/1 -> Sum4/1

== system ImuCalibrator/AINS/zero velocity update/update the underlying states/update gyro G-sensitivity ==
  In1 : Inport
  Enable : EnablePort
  Data Store Read7 : DataStoreRead  DataStoreName=Ggyr
  Data Store Write7 : DataStoreWrite  DataStoreName=Ggyr
  Reshape1 : Reshape  OutputDimensionality=Customize  OutputDimensions=[3,3]
  Sum6 : Sum  Inputs=++|
  wires:
  Sum6/1 -> Data Store Write7/1
  In1/1 -> Reshape1/1
  Reshape1/1 -> Sum6/1
  Data Store Read7/1 -> Sum6/2

== system ImuCalibrator/AINS/zero velocity update/update the underlying states/update gyro SFMA ==
  In1 : Inport
  Enable : EnablePort
  " LU Inverse1" : dspinverses/ LU Inverse
      settings: SourceProductName=DSP System Toolbox
  Bias1 : Bias  Bias=eye(3)
  Data Store Read7 : DataStoreRead  DataStoreName=Mgyr
  Data Store Write7 : DataStoreWrite  DataStoreName=Mgyr
  Data Store Write8 : DataStoreWrite  DataStoreName=IplusMinv_gyr
  Reshape1 : Reshape  OutputDimensionality=Customize  OutputDimensions=[3,3]
  Sum6 : Sum  Inputs=++|
  wires:
  Sum6/1 -> Bias1/1, Data Store Write7/1
  In1/1 -> Reshape1/1
  Reshape1/1 -> Sum6/1
  Data Store Read7/1 -> Sum6/2
  Bias1/1 -> " LU Inverse1"/1
  " LU Inverse1"/1 -> Data Store Write8/1

== matlab function ImuCalibrator/AINS/INS/MATLAB Function2 ==
  data: Cbn input; Cbn_new output; w input; dt input
function Cbn_new = update_dcm(Cbn, w, dt)

% Update attitude according to TW p.312 approximated to sixth order

rot=w*dt;
rot_norm=norm(rot);
sr_a=1-(rot_norm^2/6)+(rot_norm^4/120);
sr_b=(1/2)-(rot_norm^2/24)+(rot_norm^4/720);
mx_a=eye(3)+sr_a*skew(rot)+sr_b*skew(rot)*skew(rot);

Cbn_new=Cbn*mx_a;


function res=skew(inp_vr)
res=[0 			-inp_vr(3)	inp_vr(2); ...
     inp_vr(3)	0			-inp_vr(1);...
	 -inp_vr(2)	inp_vr(1)	0];

== matlab function ImuCalibrator/AINS/report output/MATLAB Function3 ==
  data: Cbn input; eul output size=[3,1]
function eul = dcm2euler(Cbn)

%DCM is Cbn (transforms vectors from b to n)
%eul defined as zyx sequence (yaw,pitch,roll),  but listed in
%roll,pitch,yaw order


pitch=asin(-Cbn(3,1));  %pitch is assumed to be [-pi pi]. singular at pi. use ad-hoc methods to remedy this deficiency
roll=atan2(Cbn(3,2), Cbn(3,3));
heading = atan2(Cbn(2,1), Cbn(1,1));
eul=[roll;pitch;heading];

== matlab function ImuCalibrator/AINS/gravity meas update/update the Cbn and b_g with the errors/MATLAB Function ==
  data: inp_vr input; res output
function res=skew(inp_vr)
res=[0 			-inp_vr(3)	inp_vr(2); ...
     inp_vr(3)	0			-inp_vr(1);...
	 -inp_vr(2)	inp_vr(1)	0];

== matlab function ImuCalibrator/AINS/gravity meas update/MATLAB Function1 ==
  data: S output; P input; K output; H input; R input
function [S,K] = calcKalmanGain(P, H, R)

PHT = P*H';
S = H*PHT + R;
K = PHT/S;

== matlab function ImuCalibrator/AINS/MATLAB Function ==
  data: w input; stilltime output; f input; Dt input; favgs output; wavgs output
function [stilltime, favgs, wavgs] = update_stilltime(w, f, Dt)

persistent stillt wavg favg stillcycles wsigmas fsigmas;

if isempty(wavg)
    stillt = 0;
    stillcycles = 0;
    wavg = w;
    favg = f;
    wsigmas = 0.01*[1;1;1];
    fsigmas = 0.2*[1;1;1];
end

if all(abs(f-favg) < 3*fsigmas) && all(abs(w-wavg) < 3*wsigmas)  % increment the stilltimes
    stillt = stillt + Dt;
    stillcycles = stillcycles + 1;
%     % simple recursive mean (weighting all the samples equally):
%     wavg = ((stillcycles-1)*wavg + w)/stillcycles;
%     favg = ((stillcycles-1)*favg + f)/stillcycles;

%     % recursive mean with each sample weighted by the stillcycles when it came in:
%     wavg = ((stillcycles-1)*wavg + 2*w)/(stillcycles+1);
%     favg = ((stillcycles-1)*favg + 2*f)/(stillcycles+1);

    % start with stilltime weighting and switch back to simple recursive mean after 1 second to reduce noise:
    if stillt < 1
        wavg = ((stillcycles-1)*wavg + 2*w)/(stillcycles+1);
        favg = ((stillcycles-1)*favg + 2*f)/(stillcycles+1);
    else
        wavg = ((stillcycles-1)*wavg + w)/stillcycles;
        favg = ((stillcycles-1)*favg + f)/stillcycles;
    end        
else  %reset stilltime
    stillt = 0;
    stillcycles = 0;
    wavg = w;
    favg = f;
end    

stilltime = stillt;
favgs = favg;
wavgs = wavg;
